simulink model "Ex2_PowerFlow_Original_No_SVC_Simulink"  (R2019a)
settings: Solver=VariableStepAuto  StartTime=0.0  StopTime=10.0  RelTol=1e-3
libraries: powerlib x40
settings Model: Creator=USUARIO  LastModifiedBy=USUARIO

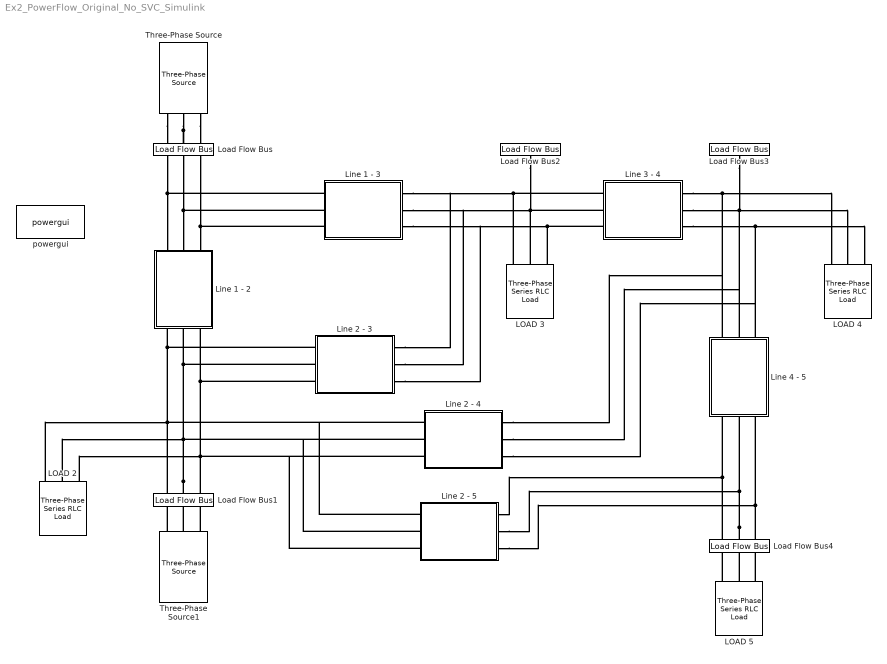
== system Ex2_PowerFlow_Original_No_SVC_Simulink ==
  LOAD 2 : powerlib/Elements/Three-Phase Series RLC Load  LConnTagsString=A|B|C  Configuration=Y (grounded)  NominalVoltage=(10000)*1  Vabc=[1e3 1e3 1e3]  Vabcp=[1e3 1e3 1e3]  NominalFrequency=60  UnbalancedPower=off  ActivePower=20e6  InductivePower=10e6  CapacitivePower=0  Pabc=[10e3 9e3 11e3]  QLabc=[100 90 110]  QCabc=[100 90 110]  Pabcp=[10e3 9e3 11e3]  QLabcp=[100 90 110]  QCabcp=[100 90 110]  Measurements=None  LoadType=constant PQ
      settings: SourceProductName=Simscape Electrical
  LOAD 3 : powerlib/Elements/Three-Phase Series RLC Load  LConnTagsString=A|B|C  Configuration=Y (grounded)  NominalVoltage=(10000)*0.987248  Vabc=[1e3 1e3 1e3]  Vabcp=[1e3 1e3 1e3]  NominalFrequency=60  UnbalancedPower=off  ActivePower=45e6  InductivePower=15e6  CapacitivePower=0  Pabc=[10e3 9e3 11e3]  QLabc=[100 90 110]  QCabc=[100 90 110]  Pabcp=[10e3 9e3 11e3]  QLabcp=[100 90 110]  QCabcp=[100 90 110]  Measurements=None  LoadType=constant PQ
      settings: SourceProductName=Simscape Electrical
  LOAD 4 : powerlib/Elements/Three-Phase Series RLC Load  LConnTagsString=A|B|C  Configuration=Y (grounded)  NominalVoltage=(10000)*0.984133  Vabc=[1e3 1e3 1e3]  Vabcp=[1e3 1e3 1e3]  NominalFrequency=60  UnbalancedPower=off  ActivePower=40e6  InductivePower=5e6  CapacitivePower=0  Pabc=[10e3 9e3 11e3]  QLabc=[100 90 110]  QCabc=[100 90 110]  Pabcp=[10e3 9e3 11e3]  QLabcp=[100 90 110]  QCabcp=[100 90 110]  Measurements=None  LoadType=constant PQ
      settings: SourceProductName=Simscape Electrical
  LOAD 5 : powerlib/Elements/Three-Phase Series RLC Load  LConnTagsString=A|B|C  Configuration=Y (grounded)  NominalVoltage=(10000)*0.971697  Vabc=[1e3 1e3 1e3]  Vabcp=[1e3 1e3 1e3]  NominalFrequency=60  UnbalancedPower=off  ActivePower=60e6  InductivePower=10e6  CapacitivePower=0  Pabc=[10e3 9e3 11e3]  QLabc=[100 90 110]  QCabc=[100 90 110]  Pabcp=[10e3 9e3 11e3]  QLabcp=[100 90 110]  QCabcp=[100 90 110]  Measurements=None  LoadType=constant PQ
      settings: SourceProductName=Simscape Electrical
  "Line 1 - 2 " : Subsystem  mask{F=60, R=0.02, XL=0.06, B=0.03}
      mask prompts: F "Frequency"; R "Resistance"; XL "Reactance"; B "Susceptance"
      mask Display: disp('Line')
  Line 1 - 3 : Subsystem  mask{F=60, R=0.08, XL=0.24, B=0.025}
      mask prompts: F "Frequency"; R "Resistance"; XL "Reactance"; B "Susceptance"
      mask Display: disp('Line')
  Line 2 - 3 : Subsystem  mask{F=60, R=0.06, XL=0.18, B=0.02}
      mask prompts: F "Frequency"; R "Resistance"; XL "Reactance"; B "Susceptance"
      mask Display: disp('Line')
  Line 2 - 4 : Subsystem  mask{F=60, R=0.06, XL=0.18, B=0.02}
      mask prompts: F "Frequency"; R "Resistance"; XL "Reactance"; B "Susceptance"
      mask Display: disp('Line')
  Line 2 - 5 : Subsystem  mask{F=60, R=0.04, XL=0.12, B=0.015}
      mask prompts: F "Frequency"; R "Resistance"; XL "Reactance"; B "Susceptance"
      mask Display: disp('Line')
  Line 3 - 4 : Subsystem  mask{F=60, R=0.01, XL=0.03, B=0.01}
      mask prompts: F "Frequency"; R "Resistance"; XL "Reactance"; B "Susceptance"
      mask Display: disp('Line')
  Line 4 - 5 : Subsystem  mask{F=60, R=0.08, XL=0.24, B=0.025}
      mask prompts: F "Frequency"; R "Resistance"; XL "Reactance"; B "Susceptance"
      mask Display: disp('Line')
  Load Flow Bus : powerlib/Measurements/Load Flow Bus  LConnTagsString=a  Phases=single  Connectors=on one side  ID=BUS_1  Vbase=10e3  Vref=1.06  Vangle=0  VLF=1.06  VLFb=1  VLFc=1  angleLF=0  angleLFb=0  angleLFc=0
      settings: SourceProductName=Simscape Electrical
  Load Flow Bus1 : powerlib/Measurements/Load Flow Bus  LConnTagsString=a  Phases=single  Connectors=on one side  ID=BUS_2  Vbase=10e3  Vref=1  Vangle=0  VLF=1  VLFb=1  VLFc=1  angleLF=-2.061  angleLFb=0  angleLFc=0
      settings: SourceProductName=Simscape Electrical
  Load Flow Bus2 : powerlib/Measurements/Load Flow Bus  LConnTagsString=a  Phases=single  Connectors=on one side  ID=BUS_3  Vbase=10e3  Vref=1.03  Vangle=0  VLF=0.9872  VLFb=1  VLFc=1  angleLF=-4.637  angleLFb=0  angleLFc=0
      settings: SourceProductName=Simscape Electrical
  Load Flow Bus3 : powerlib/Measurements/Load Flow Bus  LConnTagsString=a  Phases=single  Connectors=on one side  ID=BUS_4  Vbase=10e3  Vref=1  Vangle=0  VLF=0.9841  VLFb=1  VLFc=1  angleLF=-4.957  angleLFb=0  angleLFc=0
      settings: SourceProductName=Simscape Electrical
  Load Flow Bus4 : powerlib/Measurements/Load Flow Bus  LConnTagsString=a  Phases=single  Connectors=on one side  ID=BUS_5  Vbase=10e3  Vref=1  Vangle=0  VLF=0.9717  VLFb=1  VLFc=1  angleLF=-5.765  angleLFb=0  angleLFc=0
      settings: SourceProductName=Simscape Electrical
  Three-Phase Source : powerlib/Electrical Sources/Three-Phase Source  InternalConnection=Yg  VoltagePhases=off  Voltage=(10000)*1.06  PhaseAngle=0  Voltage_phases=[25e3 25e3 25e3]/sqrt(3)  PhaseAngles_phases=[0 -120 +120]  Frequency=60  NonIdealSource=off  SpecifyImpedance=off  Resistance=0.8929  Inductance=16.58e-3  ShortCircuitLevel=100e6  BaseVoltage=25e3  XRratio=7  BusType=swing  Pref=10e3  Qref=0  Prefabc=[10e3, 10e3, 10e3]  Qrefabc=[0, 0, 0]  Qmin=-inf  Qmax=inf
      settings: SourceProductName=Simscape Electrical
  Three-Phase Source1 : powerlib/Electrical Sources/Three-Phase Source  InternalConnection=Yg  VoltagePhases=off  Voltage=(10000)*1  PhaseAngle=-2.0612  Voltage_phases=[25e3 25e3 25e3]/sqrt(3)  PhaseAngles_phases=[0 -120 +120]  Frequency=60  NonIdealSource=off  SpecifyImpedance=off  Resistance=0.8929  Inductance=16.58e-3  ShortCircuitLevel=100e6  BaseVoltage=25e3  XRratio=7  BusType=PV  Pref=40e6  Qref=0  Prefabc=[10e3, 10e3, 10e3]  Qrefabc=[0, 0, 0]  Qmin=-inf  Qmax=inf
      settings: SourceProductName=Simscape Electrical
  powergui : powerlib/powergui  Priority=1  SimulationMode=Continuous  SampleTime=50e-6  frequency=60  Iterations=50  frequencyindice=60  Pbase=100e6  ErrMax=0.0001  UnitsV=kV  UnitsW=MW  buscounter=0  FunctionMessages=off  echomessages=off  EnableUseOfTLC=off  CurrentSourceSwitches=off  DisableSnubberDevices=off  DisableRonSwitches=off  DisableVfSwitches=off  DisplayEquations=off  AutomaticDiscreteSolvers=off  SolverType=Tustin/Backward Euler (TBE)  Interpol=off  ExternalGateDelay=off  methode=off  Ts=100  x0status=blocks  SPID=on  SwTol=0  HookPort=off  NonlinearTolerance=0  nMaxIteration=15  ContinueOnMaxIteration=off  RestoreLinks=warning  ResistiveCurrentMeasurement=off  Frange=[0:2:500]  Ylog=off  Xlog=on  ShowGrid=off  save=off  variable=ZData  structure=0  ZoomFFT=off  StartTime=0.0  cycles=1  DisplayStyle=1  fundamental=60  FreqAxis=off  MaxFrequency=1000  frequencyindicesteady=1  RmsSteady=1  display=off
      settings: SourceProductName=Simscape Electrical
  connections:
  Three-Phase Source1/RConn1 -- LOAD 2/LConn1 -- Line 2 - 5/LConn1 -- Line 2 - 4/LConn1 -- "Line 1 - 2 "/RConn1 -- Line 2 - 3/LConn1
  Three-Phase Source1/RConn2 -- LOAD 2/LConn2 -- "Line 1 - 2 "/RConn2 -- Line 2 - 3/LConn2 -- Line 2 - 4/LConn2 -- Line 2 - 5/LConn2 -- Load Flow Bus1/LConn1
  Three-Phase Source1/RConn3 -- LOAD 2/LConn3 -- "Line 1 - 2 "/RConn3 -- Line 2 - 3/LConn3 -- Line 2 - 4/LConn3 -- Line 2 - 5/LConn3
  Three-Phase Source/RConn1 -- Line 1 - 3/LConn1 -- "Line 1 - 2 "/LConn1
  Three-Phase Source/RConn2 -- Load Flow Bus/LConn1 -- Line 1 - 3/LConn2 -- "Line 1 - 2 "/LConn2
  Three-Phase Source/RConn3 -- Line 1 - 3/LConn3 -- "Line 1 - 2 "/LConn3
  LOAD 3/LConn1 -- Line 3 - 4/LConn1 -- Line 2 - 3/RConn1 -- Line 1 - 3/RConn1
  LOAD 3/LConn2 -- Line 3 - 4/LConn2 -- Load Flow Bus2/LConn1 -- Line 2 - 3/RConn2 -- Line 1 - 3/RConn2
  LOAD 3/LConn3 -- Line 3 - 4/LConn3 -- Line 2 - 3/RConn3 -- Line 1 - 3/RConn3
  Line 3 - 4/RConn1 -- Line 4 - 5/LConn1 -- Line 2 - 4/RConn1 -- LOAD 4/LConn1
  Line 3 - 4/RConn2 -- LOAD 4/LConn2 -- Load Flow Bus3/LConn1 -- Line 4 - 5/LConn2 -- Line 2 - 4/RConn2
  Line 3 - 4/RConn3 -- Line 2 - 4/RConn3 -- Line 4 - 5/LConn3 -- LOAD 4/LConn3
  LOAD 5/LConn1 -- Line 2 - 5/RConn1 -- Line 4 - 5/RConn1
  LOAD 5/LConn2 -- Load Flow Bus4/LConn1 -- Line 2 - 5/RConn2 -- Line 4 - 5/RConn2
  LOAD 5/LConn3 -- Line 2 - 5/RConn3 -- Line 4 - 5/RConn3

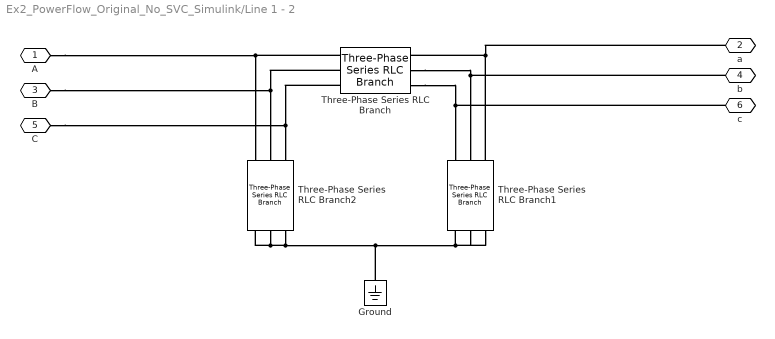
== system Ex2_PowerFlow_Original_No_SVC_Simulink/Line 1 - 2  ==
  Ground : powerlib/Elements/Ground  LConnTagsString=a
      settings: SourceProductName=Simscape Electrical
  Three-Phase Series RLC Branch : powerlib/Elements/Three-Phase Series RLC Branch  LConnTagsString=A|B|C  RConnTagsString=A|B|C  BranchType=RL  Resistance=R  Inductance=XL/(2*pi*F)  Capacitance=0  Measurements=None
      settings: SourceProductName=Simscape Electrical
  Three-Phase Series RLC Branch1 : powerlib/Elements/Three-Phase Series RLC Branch  LConnTagsString=A|B|C  RConnTagsString=A|B|C  BranchType=C  Resistance=0  Inductance=0  Capacitance=B/(2*pi*F)  Measurements=None
      settings: SourceProductName=Simscape Electrical
  Three-Phase Series RLC Branch2 : powerlib/Elements/Three-Phase Series RLC Branch  LConnTagsString=A|B|C  RConnTagsString=A|B|C  BranchType=C  Resistance=0  Inductance=0  Capacitance=B/(2*pi*F)  Measurements=None
      settings: SourceProductName=Simscape Electrical
  A : PMIOPort  Side=Left
  a : PMIOPort  Port=2  Side=Right
  B : PMIOPort  Port=3  Side=Left
  b : PMIOPort  Port=4  Side=Right
  C : PMIOPort  Port=5  Side=Left
  c : PMIOPort  Port=6  Side=Right
  connections:
  Three-Phase Series RLC Branch/RConn3 -- c/RConn1 -- Three-Phase Series RLC Branch1/LConn1
  Three-Phase Series RLC Branch2/RConn3 -- Ground/LConn1 -- Three-Phase Series RLC Branch1/RConn3 -- Three-Phase Series RLC Branch1/RConn2 -- Three-Phase Series RLC Branch1/RConn1 -- Three-Phase Series RLC Branch2/RConn2 -- Three-Phase Series RLC Branch2/RConn1
  Three-Phase Series RLC Branch/LConn3 -- C/RConn1 -- Three-Phase Series RLC Branch2/LConn3
  Three-Phase Series RLC Branch1/LConn3 -- a/RConn1 -- Three-Phase Series RLC Branch/RConn1
  Three-Phase Series RLC Branch/RConn2 -- b/RConn1 -- Three-Phase Series RLC Branch1/LConn2
  Three-Phase Series RLC Branch/LConn2 -- B/RConn1 -- Three-Phase Series RLC Branch2/LConn2
  Three-Phase Series RLC Branch/LConn1 -- A/RConn1 -- Three-Phase Series RLC Branch2/LConn1

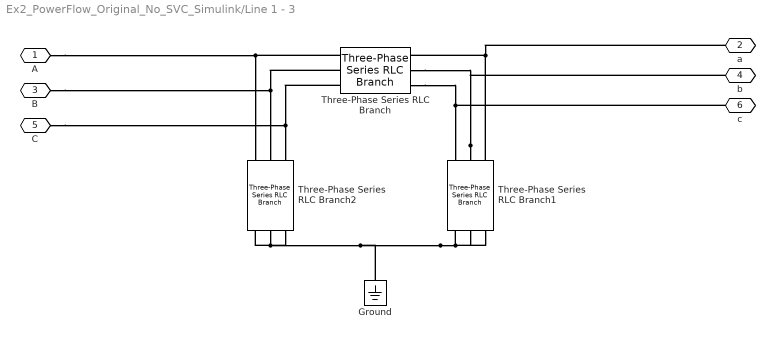
== system Ex2_PowerFlow_Original_No_SVC_Simulink/Line 1 - 3 ==
  Ground : powerlib/Elements/Ground  LConnTagsString=a
      settings: SourceProductName=Simscape Electrical
  Three-Phase Series RLC Branch : powerlib/Elements/Three-Phase Series RLC Branch  LConnTagsString=A|B|C  RConnTagsString=A|B|C  BranchType=RL  Resistance=R  Inductance=XL/(2*pi*F)  Capacitance=0  Measurements=None
      settings: SourceProductName=Simscape Electrical
  Three-Phase Series RLC Branch1 : powerlib/Elements/Three-Phase Series RLC Branch  LConnTagsString=A|B|C  RConnTagsString=A|B|C  BranchType=C  Resistance=0  Inductance=0  Capacitance=B/(2*pi*F)  Measurements=None
      settings: SourceProductName=Simscape Electrical
  Three-Phase Series RLC Branch2 : powerlib/Elements/Three-Phase Series RLC Branch  LConnTagsString=A|B|C  RConnTagsString=A|B|C  BranchType=C  Resistance=0  Inductance=0  Capacitance=B/(2*pi*F)  Measurements=None
      settings: SourceProductName=Simscape Electrical
  A : PMIOPort  Side=Left
  a : PMIOPort  Port=2  Side=Right
  B : PMIOPort  Port=3  Side=Left
  b : PMIOPort  Port=4  Side=Right
  C : PMIOPort  Port=5  Side=Left
  c : PMIOPort  Port=6  Side=Right
  connections:
  Three-Phase Series RLC Branch/RConn3 -- Three-Phase Series RLC Branch1/LConn1 -- c/RConn1
  Three-Phase Series RLC Branch2/RConn2 -- Three-Phase Series RLC Branch2/RConn1 -- Three-Phase Series RLC Branch2/RConn3 -- Three-Phase Series RLC Branch1/RConn3 -- Three-Phase Series RLC Branch1/RConn2 -- Three-Phase Series RLC Branch1/RConn1 -- Ground/LConn1
  Three-Phase Series RLC Branch/LConn3 -- Three-Phase Series RLC Branch2/LConn3 -- C/RConn1
  Three-Phase Series RLC Branch1/LConn3 -- Three-Phase Series RLC Branch/RConn1 -- a/RConn1
  Three-Phase Series RLC Branch1/LConn2 -- Three-Phase Series RLC Branch/RConn2 -- b/RConn1
  Three-Phase Series RLC Branch/LConn2 -- Three-Phase Series RLC Branch2/LConn2 -- B/RConn1
  Three-Phase Series RLC Branch/LConn1 -- Three-Phase Series RLC Branch2/LConn1 -- A/RConn1

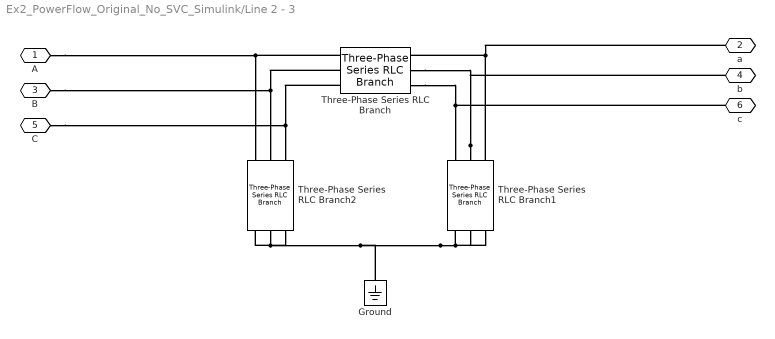
== system Ex2_PowerFlow_Original_No_SVC_Simulink/Line 2 - 3 ==
  Ground : powerlib/Elements/Ground  LConnTagsString=a
      settings: SourceProductName=Simscape Electrical
  Three-Phase Series RLC Branch : powerlib/Elements/Three-Phase Series RLC Branch  LConnTagsString=A|B|C  RConnTagsString=A|B|C  BranchType=RL  Resistance=R  Inductance=XL/(2*pi*F)  Capacitance=0  Measurements=None
      settings: SourceProductName=Simscape Electrical
  Three-Phase Series RLC Branch1 : powerlib/Elements/Three-Phase Series RLC Branch  LConnTagsString=A|B|C  RConnTagsString=A|B|C  BranchType=C  Resistance=0  Inductance=0  Capacitance=B/(2*pi*F)  Measurements=None
      settings: SourceProductName=Simscape Electrical
  Three-Phase Series RLC Branch2 : powerlib/Elements/Three-Phase Series RLC Branch  LConnTagsString=A|B|C  RConnTagsString=A|B|C  BranchType=C  Resistance=0  Inductance=0  Capacitance=B/(2*pi*F)  Measurements=None
      settings: SourceProductName=Simscape Electrical
  A : PMIOPort  Side=Left
  a : PMIOPort  Port=2  Side=Right
  B : PMIOPort  Port=3  Side=Left
  b : PMIOPort  Port=4  Side=Right
  C : PMIOPort  Port=5  Side=Left
  c : PMIOPort  Port=6  Side=Right
  connections:
  Three-Phase Series RLC Branch/RConn3 -- Three-Phase Series RLC Branch1/LConn1 -- c/RConn1
  Three-Phase Series RLC Branch2/RConn2 -- Three-Phase Series RLC Branch2/RConn1 -- Three-Phase Series RLC Branch2/RConn3 -- Three-Phase Series RLC Branch1/RConn3 -- Three-Phase Series RLC Branch1/RConn2 -- Three-Phase Series RLC Branch1/RConn1 -- Ground/LConn1
  Three-Phase Series RLC Branch/LConn3 -- Three-Phase Series RLC Branch2/LConn3 -- C/RConn1
  Three-Phase Series RLC Branch1/LConn3 -- Three-Phase Series RLC Branch/RConn1 -- a/RConn1
  Three-Phase Series RLC Branch1/LConn2 -- Three-Phase Series RLC Branch/RConn2 -- b/RConn1
  Three-Phase Series RLC Branch/LConn2 -- Three-Phase Series RLC Branch2/LConn2 -- B/RConn1
  Three-Phase Series RLC Branch/LConn1 -- Three-Phase Series RLC Branch2/LConn1 -- A/RConn1

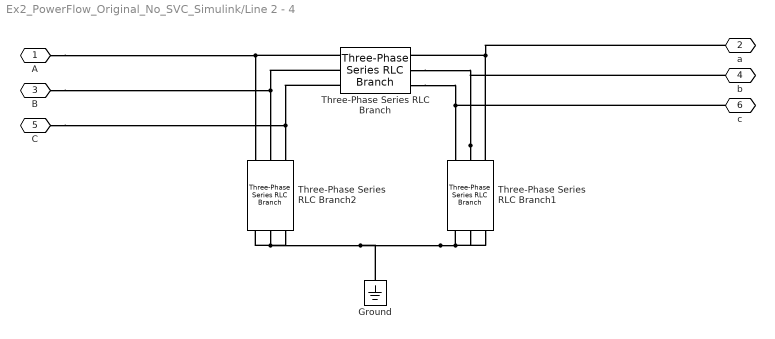
== system Ex2_PowerFlow_Original_No_SVC_Simulink/Line 2 - 4 ==
  Ground : powerlib/Elements/Ground  LConnTagsString=a
      settings: SourceProductName=Simscape Electrical
  Three-Phase Series RLC Branch : powerlib/Elements/Three-Phase Series RLC Branch  LConnTagsString=A|B|C  RConnTagsString=A|B|C  BranchType=RL  Resistance=R  Inductance=XL/(2*pi*F)  Capacitance=0  Measurements=None
      settings: SourceProductName=Simscape Electrical
  Three-Phase Series RLC Branch1 : powerlib/Elements/Three-Phase Series RLC Branch  LConnTagsString=A|B|C  RConnTagsString=A|B|C  BranchType=C  Resistance=0  Inductance=0  Capacitance=B/(2*pi*F)  Measurements=None
      settings: SourceProductName=Simscape Electrical
  Three-Phase Series RLC Branch2 : powerlib/Elements/Three-Phase Series RLC Branch  LConnTagsString=A|B|C  RConnTagsString=A|B|C  BranchType=C  Resistance=0  Inductance=0  Capacitance=B/(2*pi*F)  Measurements=None
      settings: SourceProductName=Simscape Electrical
  A : PMIOPort  Side=Left
  a : PMIOPort  Port=2  Side=Right
  B : PMIOPort  Port=3  Side=Left
  b : PMIOPort  Port=4  Side=Right
  C : PMIOPort  Port=5  Side=Left
  c : PMIOPort  Port=6  Side=Right
  connections:
  Three-Phase Series RLC Branch/RConn3 -- Three-Phase Series RLC Branch1/LConn1 -- c/RConn1
  Three-Phase Series RLC Branch2/RConn2 -- Three-Phase Series RLC Branch2/RConn1 -- Three-Phase Series RLC Branch2/RConn3 -- Three-Phase Series RLC Branch1/RConn3 -- Three-Phase Series RLC Branch1/RConn2 -- Three-Phase Series RLC Branch1/RConn1 -- Ground/LConn1
  Three-Phase Series RLC Branch/LConn3 -- Three-Phase Series RLC Branch2/LConn3 -- C/RConn1
  Three-Phase Series RLC Branch1/LConn3 -- Three-Phase Series RLC Branch/RConn1 -- a/RConn1
  Three-Phase Series RLC Branch1/LConn2 -- Three-Phase Series RLC Branch/RConn2 -- b/RConn1
  Three-Phase Series RLC Branch/LConn2 -- Three-Phase Series RLC Branch2/LConn2 -- B/RConn1
  Three-Phase Series RLC Branch/LConn1 -- Three-Phase Series RLC Branch2/LConn1 -- A/RConn1

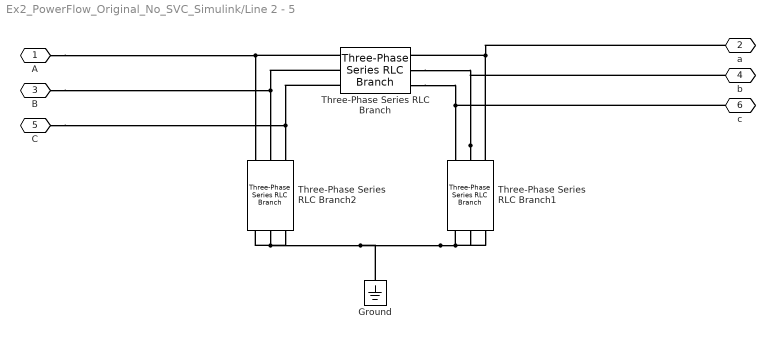
== system Ex2_PowerFlow_Original_No_SVC_Simulink/Line 2 - 5 ==
  Ground : powerlib/Elements/Ground  LConnTagsString=a
      settings: SourceProductName=Simscape Electrical
  Three-Phase Series RLC Branch : powerlib/Elements/Three-Phase Series RLC Branch  LConnTagsString=A|B|C  RConnTagsString=A|B|C  BranchType=RL  Resistance=R  Inductance=XL/(2*pi*F)  Capacitance=0  Measurements=None
      settings: SourceProductName=Simscape Electrical
  Three-Phase Series RLC Branch1 : powerlib/Elements/Three-Phase Series RLC Branch  LConnTagsString=A|B|C  RConnTagsString=A|B|C  BranchType=C  Resistance=0  Inductance=0  Capacitance=B/(2*pi*F)  Measurements=None
      settings: SourceProductName=Simscape Electrical
  Three-Phase Series RLC Branch2 : powerlib/Elements/Three-Phase Series RLC Branch  LConnTagsString=A|B|C  RConnTagsString=A|B|C  BranchType=C  Resistance=0  Inductance=0  Capacitance=B/(2*pi*F)  Measurements=None
      settings: SourceProductName=Simscape Electrical
  A : PMIOPort  Side=Left
  a : PMIOPort  Port=2  Side=Right
  B : PMIOPort  Port=3  Side=Left
  b : PMIOPort  Port=4  Side=Right
  C : PMIOPort  Port=5  Side=Left
  c : PMIOPort  Port=6  Side=Right
  connections:
  Three-Phase Series RLC Branch/RConn3 -- Three-Phase Series RLC Branch1/LConn1 -- c/RConn1
  Three-Phase Series RLC Branch2/RConn2 -- Three-Phase Series RLC Branch2/RConn1 -- Three-Phase Series RLC Branch2/RConn3 -- Three-Phase Series RLC Branch1/RConn3 -- Three-Phase Series RLC Branch1/RConn2 -- Three-Phase Series RLC Branch1/RConn1 -- Ground/LConn1
  Three-Phase Series RLC Branch/LConn3 -- Three-Phase Series RLC Branch2/LConn3 -- C/RConn1
  Three-Phase Series RLC Branch1/LConn3 -- Three-Phase Series RLC Branch/RConn1 -- a/RConn1
  Three-Phase Series RLC Branch1/LConn2 -- Three-Phase Series RLC Branch/RConn2 -- b/RConn1
  Three-Phase Series RLC Branch/LConn2 -- Three-Phase Series RLC Branch2/LConn2 -- B/RConn1
  Three-Phase Series RLC Branch/LConn1 -- Three-Phase Series RLC Branch2/LConn1 -- A/RConn1

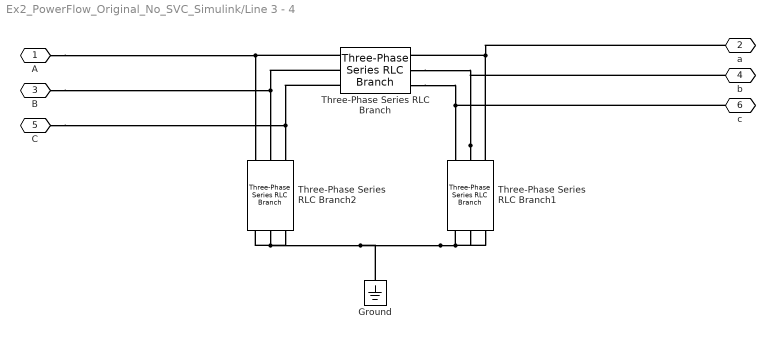
== system Ex2_PowerFlow_Original_No_SVC_Simulink/Line 3 - 4 ==
  Ground : powerlib/Elements/Ground  LConnTagsString=a
      settings: SourceProductName=Simscape Electrical
  Three-Phase Series RLC Branch : powerlib/Elements/Three-Phase Series RLC Branch  LConnTagsString=A|B|C  RConnTagsString=A|B|C  BranchType=RL  Resistance=R  Inductance=XL/(2*pi*F)  Capacitance=0  Measurements=None
      settings: SourceProductName=Simscape Electrical
  Three-Phase Series RLC Branch1 : powerlib/Elements/Three-Phase Series RLC Branch  LConnTagsString=A|B|C  RConnTagsString=A|B|C  BranchType=C  Resistance=0  Inductance=0  Capacitance=B/(2*pi*F)  Measurements=None
      settings: SourceProductName=Simscape Electrical
  Three-Phase Series RLC Branch2 : powerlib/Elements/Three-Phase Series RLC Branch  LConnTagsString=A|B|C  RConnTagsString=A|B|C  BranchType=C  Resistance=0  Inductance=0  Capacitance=B/(2*pi*F)  Measurements=None
      settings: SourceProductName=Simscape Electrical
  A : PMIOPort  Side=Left
  a : PMIOPort  Port=2  Side=Right
  B : PMIOPort  Port=3  Side=Left
  b : PMIOPort  Port=4  Side=Right
  C : PMIOPort  Port=5  Side=Left
  c : PMIOPort  Port=6  Side=Right
  connections:
  Three-Phase Series RLC Branch/RConn3 -- Three-Phase Series RLC Branch1/LConn1 -- c/RConn1
  Three-Phase Series RLC Branch2/RConn2 -- Three-Phase Series RLC Branch2/RConn1 -- Three-Phase Series RLC Branch2/RConn3 -- Three-Phase Series RLC Branch1/RConn3 -- Three-Phase Series RLC Branch1/RConn2 -- Three-Phase Series RLC Branch1/RConn1 -- Ground/LConn1
  Three-Phase Series RLC Branch/LConn3 -- Three-Phase Series RLC Branch2/LConn3 -- C/RConn1
  Three-Phase Series RLC Branch1/LConn3 -- Three-Phase Series RLC Branch/RConn1 -- a/RConn1
  Three-Phase Series RLC Branch1/LConn2 -- Three-Phase Series RLC Branch/RConn2 -- b/RConn1
  Three-Phase Series RLC Branch/LConn2 -- Three-Phase Series RLC Branch2/LConn2 -- B/RConn1
  Three-Phase Series RLC Branch/LConn1 -- Three-Phase Series RLC Branch2/LConn1 -- A/RConn1

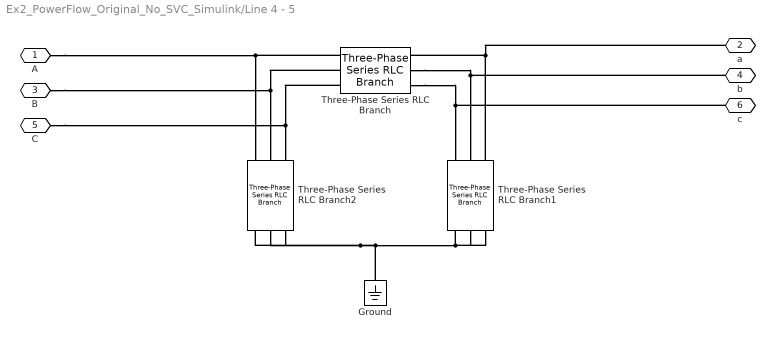
== system Ex2_PowerFlow_Original_No_SVC_Simulink/Line 4 - 5 ==
  Ground : powerlib/Elements/Ground  LConnTagsString=a
      settings: SourceProductName=Simscape Electrical
  Three-Phase Series RLC Branch : powerlib/Elements/Three-Phase Series RLC Branch  LConnTagsString=A|B|C  RConnTagsString=A|B|C  BranchType=RL  Resistance=R  Inductance=XL/(2*pi*F)  Capacitance=0  Measurements=None
      settings: SourceProductName=Simscape Electrical
  Three-Phase Series RLC Branch1 : powerlib/Elements/Three-Phase Series RLC Branch  LConnTagsString=A|B|C  RConnTagsString=A|B|C  BranchType=C  Resistance=0  Inductance=0  Capacitance=B/(2*pi*F)  Measurements=None
      settings: SourceProductName=Simscape Electrical
  Three-Phase Series RLC Branch2 : powerlib/Elements/Three-Phase Series RLC Branch  LConnTagsString=A|B|C  RConnTagsString=A|B|C  BranchType=C  Resistance=0  Inductance=0  Capacitance=B/(2*pi*F)  Measurements=None
      settings: SourceProductName=Simscape Electrical
  A : PMIOPort  Side=Left
  a : PMIOPort  Port=2  Side=Right
  B : PMIOPort  Port=3  Side=Left
  b : PMIOPort  Port=4  Side=Right
  C : PMIOPort  Port=5  Side=Left
  c : PMIOPort  Port=6  Side=Right
  connections:
  A/RConn1 -- Three-Phase Series RLC Branch2/LConn1 -- Three-Phase Series RLC Branch/LConn1
  B/RConn1 -- Three-Phase Series RLC Branch2/LConn2 -- Three-Phase Series RLC Branch/LConn2
  b/RConn1 -- Three-Phase Series RLC Branch/RConn2 -- Three-Phase Series RLC Branch1/LConn2
  a/RConn1 -- Three-Phase Series RLC Branch/RConn1 -- Three-Phase Series RLC Branch1/LConn3
  C/RConn1 -- Three-Phase Series RLC Branch2/LConn3 -- Three-Phase Series RLC Branch/LConn3
  Ground/LConn1 -- Three-Phase Series RLC Branch1/RConn1 -- Three-Phase Series RLC Branch1/RConn2 -- Three-Phase Series RLC Branch1/RConn3 -- Three-Phase Series RLC Branch2/RConn3 -- Three-Phase Series RLC Branch2/RConn1 -- Three-Phase Series RLC Branch2/RConn2
  c/RConn1 -- Three-Phase Series RLC Branch1/LConn1 -- Three-Phase Series RLC Branch/RConn3
